simulink model "TWFL_V2"  (R2025b)
settings: Solver=daessc  StartTime=0.0  StopTime=15  RelTol=1e-3
values from neighbouring files (symbols this model uses):
  g = 9.81    [model_simplified.m]    (also in robotParams.m)
  g_fork = 2*pi*3    (= 18.8495559215)    [robotParams.m]
  g_lift = 2*pi*5    (= 31.4159265359)    [robotParams.m]
  g_reac = 2*pi*1    (= 6.28318530718)    [robotParams.m]
  Kd_fork = 100    [robotParams.m]
  Kd_lift = 50    [robotParams.m]
  Kp_fork = 200    [robotParams.m]
  Kp_lift = 200    [robotParams.m]
  Lx_b = 0.3    [robotParams.m]
  Lx_m = 0.1    [robotParams.m]
  Ly_b = 0.8    [robotParams.m]
  Ly_m = 0.3    [robotParams.m]
  Lz_b = 1    [robotParams.m]
  Lz_m = 1.5    [robotParams.m]
  M_arm_motor = 5    [robotParams.m]
  M_b = 16    [robotParams.m]
  M_fork_base = 2    [robotParams.m]
  M_m = 5    [robotParams.m]
  M_tooth = 1    [robotParams.m]
  M_w = 1    [robotParams.m]
  N = 40    [ocp_arm.m]    (also in ocp_simplified.m)
  r_w = 0.2    [model_simplified.m]    (also in robotParams.m)
  T_control = 1e-3    (= 0.001)    [robotParams.m]
  t_w = 0.05    [robotParams.m]
undefined symbols (not defined in the file or in its folder): dspblkCoreblockFVToolHelper, gcbh, Mn_33, Mn_44, X, Y, Z
libraries: sm_lib x49, nesl_utility x13, simulink x9, slpidlib x1, SignalEditorBlockLib x1
(part 1 of 3)
settings Model: Creator=oj  LastModifiedBy=angel
settings DataIOCC: SaveFormat=StructureWithTime
settings OptimizationCC: LifeSpan=inf
settings DebuggingCC: UnconnectedInputMsg=warning  UnconnectedOutputMsg=warning  UnconnectedLineMsg=warning  SFExecutionAtInitializationDiag=none  ArithmeticOperatorsInVariantConditions=warning
settings HardwareCC: ProdBitPerSizeT=32.0  ProdBitPerPtrDiffT=32.0  ProdWordSize=32.0  ProdHWDeviceType=Specified
settings SFSimCC: CustomCodeUndefinedFunction=UseInterfaceOnly
settings RTWCC: GPUComputeCapability=3.5
settings CodeAppCC: StateflowObjectComments=on

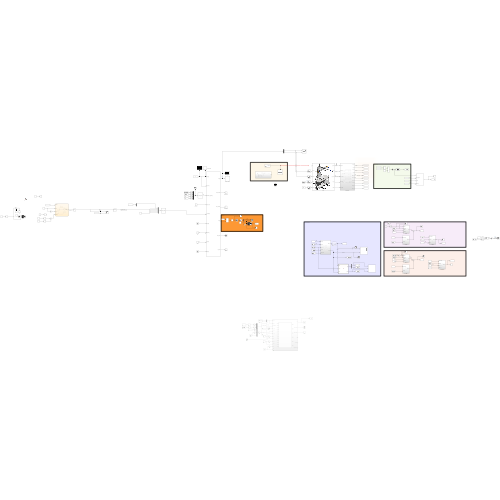
[thumbnail: Simulink's stored preview of the top-level diagram]
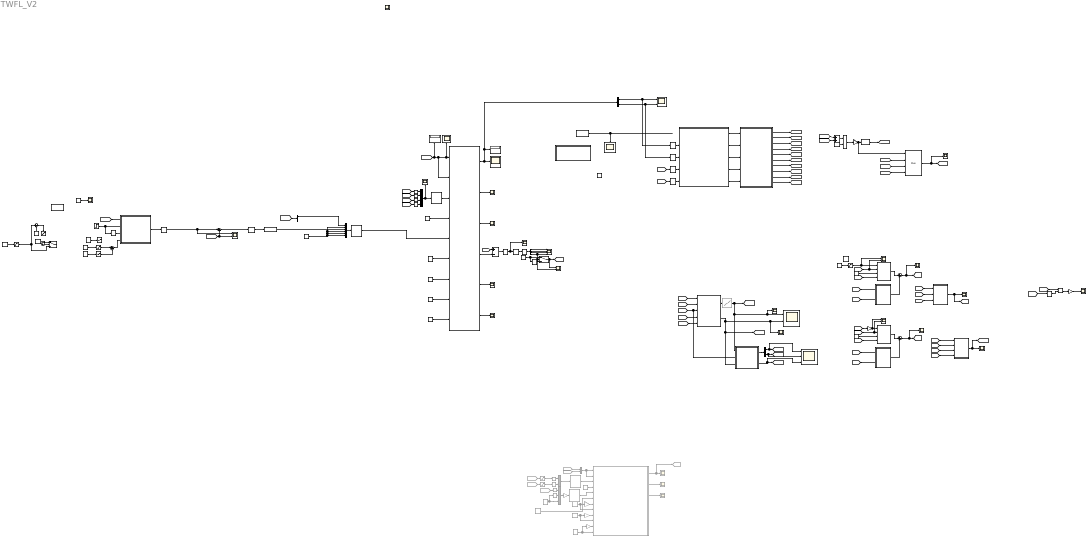
== system TWFL_V2 ==
  note: Collision
  note: CoG Estimation
  note: Calculations
  note: Disturbance
  note: FORK
  note: LIFT
  1-D Lookup Table2 : Lookup_n-D  Commented=through  NumberOfTableDimensions=1  BreakpointsForDimension1=[0:20]  Table=[0:20]  InterpMethod=Flat  InternalRulePriority=Speed  RndMeth=Simplest
  Abs : Abs  SaturateOnIntegerOverflow=off
  Abs1 : Abs  SaturateOnIntegerOverflow=off
  CPU : Scope
      settings: Description=status  ActiveDisplayYMinimum=0.0016298375  ActiveDisplayYMaximum=0.0033734625  DataLoggingVariableName=ScopeData3
  Calculations : Subsystem
  Chart : Stateflow chart  TreatAsAtomicUnit=on
  Clock1 : Clock
      settings: Decimation=9
  Constant{,16,42..43} (4 alike) : Constant  Value=0
  Constant14 : Constant
  Constant17 : Constant  Commented=on  Value=[0 0 0]
  Constant18 : Constant  Commented=on  Value=[0 0]
  Constant19 : Constant  Commented=on  Value=[pi/4; 0.5]
  Constant20 : Constant  Commented=on  Value=0
  Constant23 : Constant  Commented=on  Value=repmat([pi/4; 0.5],N-1,1)
  Constant26 : Constant  Commented=on  Value=repmat([100],N,1)
  Constant45 : Constant  Value=0.1
  Constant6 : Constant  Value=2
  Constant8 : Constant  Value=-2
  Cos : Trigonometry  Operator=cos
  Delay : Delay  DelayLength=1  InputProcessing=Columns as channels (frame based)
  Demux : Demux  Outputs=2
  Demux1 : Demux  Outputs=2
  Demux2 : Demux
  Demux4 : Demux
  Discrete Derivative : simulink/Discrete/Discrete Derivative  gainval=1.0  ICPrevScaledInput=0.0  OutMin=[]  OutMax=[]  OutDataType=fixdt(1, 16)  OutScaling=2^-10  DoSatur=off
  Discrete Derivative1 : simulink/Discrete/Discrete Derivative  gainval=1.0  ICPrevScaledInput=0.0  OutMin=[]  OutMax=[]  OutDataType=fixdt(1, 16)  OutScaling=2^-10  DoSatur=off
  Display2 : Display
  Divide : Product  Inputs=*/
  Divide1 : Product  Inputs=*/
  Fork DOB : Subsystem
  Fork RDOB : Subsystem
  From25 : From  Commented=on  GotoTag=pitch_pos
  From26 : From  Commented=on  GotoTag=dist_hat
  From5 : From  Commented=on  GotoTag=arm_pos
  From6 : From  Commented=on  GotoTag=arm_vel
  From7 : From  Commented=on  GotoTag=mass_hat
  Gain{,1,3..4} (4 alike) : Gain  Commented=on  Gain=-1
  Gain12 : Gain  Gain=1/g
  Gain18 : Gain  Gain=-1
  Gain2 : Gain  Gain=r_w
  Goto6 : Goto  Commented=on  GotoTag=torque_arm
  KKT residual : Scope
      settings: Description=status  ActiveDisplayYMinimum=-0.63612459745356664  ActiveDisplayYMaximum=2.0677690230743266  DataLoggingVariableName=ScopeData4
  Lift DOB : Subsystem
  Lift RDOB : Subsystem
  MATLAB Function1 : MATLAB Function  TreatAsAtomicUnit=on
  Mux : Mux
      settings: DisplayOption=signals
  Mux2 : Mux  Inputs=6
  Mux4 : Mux
  Mux6 : Mux  Commented=on  Inputs=2
  Mux7 : Mux  Commented=on  Inputs=2
  Mux8 : Mux  Commented=on  Inputs=3
  NOT : Logic  Operator=NOT  IconShape=distinctive  AllPortsSameDT=off  OutDataTypeStr=boolean
  NOT1 : Logic  Operator=NOT  IconShape=distinctive  AllPortsSameDT=off  OutDataTypeStr=boolean
  OCP status : Scope
      settings: Description=status  ActiveDisplayYMinimum=-0.0035735878879828986  ActiveDisplayYMaximum=2.0531825990917243
  PD fork : Subsystem
  PD lift : Subsystem
  PID Controller : slpidlib/PID Controller  Controller=PID  Form=Parallel  TimeDomain=Discrete-time  UseExternalTs=off  SampleTime=-1  IntegratorMethod=Forward Euler  FilterMethod=Forward Euler  ControllerParametersSource=internal  P=2  I=1  UseKiTs=off  D=0  UseExternalDerivativeSource=off  N=100  UseFilter=on  TunerSelectOption=Transfer Function Based (PID Tuner App)  InitialConditionSource=internal  InitialConditionForIntegrator=0  InitialConditionForFilter=0  DifferentiatorICPrevScaledInput=0  ExternalReset=none  TrackingMode=off  Kt=1  LimitOutput=off  SatLimitsSource=internal  UpperSaturationLimit=inf  LowerSaturationLimit=-inf  LinearizeAsGain=on  AntiWindupMode=none  Kb=1  LimitIntegrator=off  UpperIntegratorSaturationLimit=inf  LowerIntegratorSaturationLimit=-inf  POutMin=[]  POutMax=[]  IOutMin=[]  IOutMax=[]  DOutMin=[]  DOutMax=[]  NOutMin=[]  NOutMax=[]  SumOutMin=[]  SumOutMax=[]  SaturationOutMin=[]  SaturationOutMax=[]  PParamMin=[]  PParamMax=[]  IParamMin=[]  IParamMax=[]  DParamMin=[]  DParamMax=[]  NParamMin=[]  NParamMax=[]  KbParamMin=[]  KbParamMax=[]  KtParamMin=[]  KtParamMax=[]  KbOutMin=[]  KbOutMax=[]  KtOutMin=[]  KtOutMax=[]  IntegratorOutMin=[]  IntegratorOutMax=[]  FilterOutMin=[]  FilterOutMax=[]  SumI1OutMin=[]  SumI1OutMax=[]  SumI2OutMin=[]  SumI2OutMax=[]  SumI3OutMin=[]  SumI3OutMax=[]  SumI4OutMin=[]  SumI4OutMax=[]  SumDOutMin=[]  SumDOutMax=[]  DifferentiatorOutMin=[]  DifferentiatorOutMax=[]  FilterDiffOutCoefMin=[]  FilterDiffOutCoefMax=[]  ReciprocalOutMin=[]  ReciprocalOutMax=[]  SumDenOutMin=[]  SumDenOutMax=[]  SumNumOutMin=[]  SumNumOutMax=[]  DivideOutMin=[]  DivideOutMax=[]  UdiffTsProdOutMin=[]  UdiffTsProdOutMax=[]  NTsProdOutMin=[]  NTsProdOutMax=[]  UintegralTsProdOutMin=[]  UintegralTsProdOutMax=[]  UngainTsProdOutMin=[]  UngainTsProdOutMax=[]  ClampingZeroOutDataTypeStr=Inherit: Inherit via back propagation  ClampingZeroOutMin=[]  ClampingZeroOutMax=[]  FilterDenConstantOutDataTypeStr=Inherit: Inherit via back propagation  FilterDenConstantOutMin=[]  FilterDenConstantOutMax=[]  PCopyOutDataTypeStr=Inherit: Inherit via back propagation  PCopyOutMin=[]  PCopyOutMax=[]  NCopyOutDataTypeStr=Inherit: Inherit via back propagation  NCopyOutMin=[]  NCopyOutMax=[]  IntegratorContinuousStateAttributes=''  IntegratorStateMustResolveToSignalObject=off  IntegratorRTWStateStorageClass=Auto  FilterContinuousStateAttributes=''  FilterStateMustResolveToSignalObject=off  FilterRTWStateStorageClass=Auto  ParallelPVariant=InternalParameters  IdealPVariant=Disabled  IVariant=InternalParameters  DVariant=InternalParameters  IntegratorVariant=Discrete  SatVariant=Disabled  AWVariant=Passthrough  PCopyVariant=Disabled  TRVariant=Disabled  FdbkBlocksVariant=Forward  IdealPFdbkVariant=Disabled  SatFdbkVariant=Disabled  DerivativeFilterVariant=ForwardEulerFilter  NVariant=InternalParameters  NCopyVariant=Disabled  FilterICVariant=InternalICsFilter  IntegratorICVariant=InternalICs  ExternalResetVariant=Disabled  TRSumVariant=Passthrough  SumFdbkVariant=Disabled  SumVariant=Sum_PID  TsampFilterVariant=InternalTs  TsampNgainVariant=Passthrough  TsampIntegralVariant=Disabled_SignalSpec  ExternalSaturationOutDataTypeStr=Inherit: Same as second input  DerivativeSourceVariant=ErrorSignal  PreIntVariant=InternalPreInt
  Plant5 : Subsystem
      mask Display: image('plant.png');
  Push Button : PushButtonBlock  ButtonText=Start  ButtonType=Latch  IconOnColor=[0.0, 1.0, 0.0]  IconOffColor=[1.0, 1.0, 1.0]  IconColor=On  OffValue=0.000000
  Ramp1 : simulink/Sources/Ramp  slope=0.05  start=3  InitialOutput=0
  Ramp2 : simulink/Sources/Ramp  slope=1  start=9  InitialOutput=0
  Ramp3 : simulink/Sources/Ramp  slope=2  start=0  InitialOutput=0
  Ramp4 : simulink/Sources/Ramp  slope=1  start=1  InitialOutput=0
  Ramp5 : simulink/Sources/Ramp  slope=1  start=10  InitialOutput=0
  Ramp6 : simulink/Sources/Ramp  slope=1  start=5  InitialOutput=0
  Rate Transition{,1..3} (4 alike) : RateTransition  OutPortSampleTime=T_control
  S-Function1 : S-Function  FunctionName=acados_solver_sfunction_model_simplified  SFunctionDeploymentMode=off  EnableBusSupport=off
      mask Display:
      | % from the make_sfun file
      | global sfun_input_names sfun_output_names
      | for i = 1:length(sfun_input_names)
      | 	port_label('input', i, sfun_input_names{i})
      | end
      | for i = 1:length(sfun_output_names)
      | 	port_label('output', i, sfun_output_names{i})
      | end
  S-Function2 : S-Function  FunctionName=repmat_sfun  Parameters=N+1  SFunctionDeploymentMode=off  EnableBusSupport=off
  S-Function3 : S-Function  Commented=on  FunctionName=repmat_sfun  Parameters=N+1  SFunctionDeploymentMode=off  EnableBusSupport=off
  S-Function4 : S-Function  Commented=on  FunctionName=repmat_sfun  Parameters=N-1  SFunctionDeploymentMode=off  EnableBusSupport=off
  S-Function5 : S-Function  FunctionName=repmat_sfun  Parameters=N-1  SFunctionDeploymentMode=off  EnableBusSupport=off
  SQP iter : Scope
      settings: Description=status  ActiveDisplayYMinimum=-11.826905175074671  ActiveDisplayYMaximum=55.703090781193573  DataLoggingVariableName=ScopeData5
  Saturation : Saturate  UpperLimit=5  LowerLimit=0
  Saturation1 : Saturate
  Saturation2 : Saturate  UpperLimit=.25
  Saturation3 : Saturate
  Saturation4 : Saturate  Commented=on  UpperLimit=20  LowerLimit=0
  Saturation5 : Saturate  Commented=on  UpperLimit=0.6  LowerLimit=0.2
  Saturation6 : Saturate  UpperLimit=1  LowerLimit=0
  Saturation7 : Saturate  UpperLimit=1  LowerLimit=0
  Scope control : Scope
      settings: ActiveDisplayYMinimum=-179.76344795838239  ActiveDisplayYMaximum=28.261944980460278  DataLoggingVariableName=ScopeData6
  Scope state1 : Scope
      settings: ActiveDisplayYMinimum=-2.6646698598678142  ActiveDisplayYMaximum=0.29678375248917371  DataLoggingVariableName=ScopeData9
  Scope1 : Scope  NumInputPorts=4
      settings: ActiveDisplayYMinimum=-96.781255241402022  ActiveDisplayYMaximum=871.03129768928852  DataLoggingVariableName=ScopeData26
  Scope{2..3,10,12,17,26} (6 alike) : Scope  NumInputPorts=2
      Scope10 settings: ActiveDisplayYMinimum=-0.12499999999999997  ActiveDisplayYMaximum=1.125  DataLoggingVariableName=ScopeData28
      Scope12 settings: ActiveDisplayYMinimum=-1  ActiveDisplayYMaximum=1  DataLoggingVariableName=ScopeData31
      Scope17 settings: ActiveDisplayYMinimum=-1  ActiveDisplayYMaximum=1  DataLoggingVariableName=ScopeData35
      Scope2 settings: ActiveDisplayYMinimum=-4.7265728175160966  ActiveDisplayYMaximum=6.508300219679283  DataLoggingVariableName=ScopeData2
      Scope26 settings: ActiveDisplayYMinimum=0.31875  ActiveDisplayYMaximum=0.63125  DataLoggingVariableName=ScopeData32
      Scope3 settings: ActiveDisplayYMinimum=-12.49999999999882  ActiveDisplayYMaximum=12.499999999991127  DataLoggingVariableName=ScopeData10
  Scope{,4..7,9,11,16,18..21} (12 alike) : Scope
      Scope11 settings: ActiveDisplayYMinimum=-0.2386803915005089  ActiveDisplayYMaximum=1.7974378919712937  DataLoggingVariableName=ScopeData29
      Scope16 settings: ActiveDisplayYMinimum=-1  ActiveDisplayYMaximum=1  DataLoggingVariableName=ScopeData27
      Scope18 settings: ActiveDisplayYMinimum=-1  ActiveDisplayYMaximum=1  DataLoggingVariableName=ScopeData36
      Scope19 settings: ActiveDisplayYMinimum=-1  ActiveDisplayYMaximum=1  DataLoggingVariableName=ScopeData37
      Scope20 settings: ActiveDisplayYMinimum=74.24782414299321  ActiveDisplayYMaximum=93.660209670148674  DataLoggingVariableName=ScopeData39
      Scope21 settings: ActiveDisplayYMinimum=-1  ActiveDisplayYMaximum=1  DataLoggingVariableName=ScopeData40
      Scope4 settings: ActiveDisplayYMinimum=-125.68830085745365  ActiveDisplayYMaximum=62.810118223913989  DataLoggingVariableName=ScopeData11
      Scope5 settings: ActiveDisplayYMinimum=-7.37133327140659  ActiveDisplayYMaximum=14.471332987171895  DataLoggingVariableName=ScopeData12
      Scope6 settings: ActiveDisplayYMinimum=-0.193211762638459  ActiveDisplayYMaximum=0.32936826449448647  DataLoggingVariableName=ScopeData13
      Scope7 settings: ActiveDisplayYMinimum=-2.8032822197416674  ActiveDisplayYMaximum=3.1027732142135709  DataLoggingVariableName=ScopeData7
      Scope9 settings: ActiveDisplayYMinimum=-1  ActiveDisplayYMaximum=1  DataLoggingVariableName=ScopeData19
      Scope settings: ActiveDisplayYMinimum=-13.79726  ActiveDisplayYMaximum=10.28583
  Scope13 : Scope  Commented=on
      settings: ActiveDisplayYMinimum=-12.276347103940505  ActiveDisplayYMaximum=17.806393317198079  DataLoggingVariableName=ScopeData33
  Scope14 : Scope  Commented=on
      settings: ActiveDisplayYMinimum=-0.63087824577294693  ActiveDisplayYMaximum=5.157246754227053  DataLoggingVariableName=ScopeData34
  Scope15 : Scope  Commented=on
      settings: ActiveDisplayYMinimum=-1  ActiveDisplayYMaximum=1  DataLoggingVariableName=ScopeData38
  Scope8 : Scope  NumInputPorts=3
      settings: ActiveDisplayYMinimum=-8.2743101469477089  ActiveDisplayYMaximum=17.001393340631182  DataLoggingVariableName=ScopeData21
  Signal Generator : SignalGenerator  Units=rad/sec
  Signal Editor : SignalEditorBlockLib/Signal Editor  FileName=disturbance.mat  ActiveScenario=Scenario  ActiveSignal=Signal 1  IsBus=off  OutputBusObjectStr=Bus: BusObject  SampleTime=0  ZeroCross=off  OutputAfterFinalValue=Setting to zero  Unit=inherit  PreserveSignalName=on  ApplySigPropsToAllScenarios=on  ApplySigPropsToAllSignals=off  SignalPropertySource=Dialog parameters
  Signal Specification : SignalSpecification  OutDataTypeStr=double  Dimensions=1
  Signal Specification{1..4} (4 alike) : SignalSpecification  Dimensions=1
  Signal Specification{9..12} (4 alike) : SignalSpecification  Commented=on  Dimensions=1
  Step1 : Step  Time=5  SampleTime=0
  Subsystem : Subsystem
  Subsystem1 : Subsystem  Commented=on
  Subsystem2 : Subsystem
  Subtract : Sum  Inputs=+-
  Sum : Sum  Inputs=+|+
  Sum1 : Sum  Inputs=|+-
  Sum16 : Sum  Inputs=|++
  Sum17 : Sum  Inputs=|++
  Sum3 : Sum  Inputs=|+-
  Sum5 : Sum  Inputs=|+-
  Switch2 : Switch  Criteria=u2 > Threshold  Threshold=4.8  SaturateOnIntegerOverflow=off  InputSameDT=off
  Switch3 : Switch  Criteria=u2 > Threshold  Threshold=200  SaturateOnIntegerOverflow=off  InputSameDT=off
  lbu : Constant  Value=repmat([-10;-10],N,1)
  lbx : Constant  Value=repmat([-50; -pi/4; -3; -pi],N-1,1)
  q : Scope
      settings: ActiveDisplayYMinimum=-0.062737495046845726  ActiveDisplayYMaximum=0.56463747287082289  DataLoggingVariableName=ScopeData30
  u : Display
  ubu : Constant  Value=repmat([10;10],N,1)
  ubx : Constant  Value=repmat([500; pi/4; 5; pi],N-1,1)
  y_ref_0 : Constant  Value=zeros(1,6)
  wires:
  S-Function1/5 -> CPU/1
  S-Function1/6 -> SQP iter/1
  S-Function1/3 -> KKT residual/1
  Mux/1 -> Scope7/1, [q_0]  "x"
  S-Function1/4 -> Subtract/2
  S-Function1/2 -> OCP status/1
  S-Function1/1 -> Demux/1, u/1, Scope control/1  "u"
  lbx/1 -> S-Function1/6
  Demux/1 -> Rate Transition2/1, Scope3/1
  Calculations/1(rw_pos) -> [rw_pos]  "rw_angle"
  Calculations/3(lw_pos) -> [lw_pos]  "lw_angle"
  Calculations/5(pitch_pos) -> [pitch_pos]  "pitch_angle"
  Sum/1 -> Divide1/1
  Constant6/1 -> Divide1/2
  Divide1/1 -> Gain2/1
  Gain2/1 -> Mux/1, Discrete Derivative/1  "x"
  Discrete Derivative/1 -> [x_vel]  "x_dot"
  lbu/1 -> S-Function1/8
  ubu/1 -> S-Function1/9
  Demux/2 -> Rate Transition3/1, Scope3/2
  Mux2/1 -> S-Function5/1
  Demux2/1 -> Mux2/1
  Sum3/1 -> PID Controller/1
  Ramp3/1 -> Saturation1/1
  PID Controller/1 -> Signal Specification/1
  Signal Specification/1 -> Mux2/3
  ubx/1 -> S-Function1/7
  Ramp2/1 -> Sum5/2
  Clock1/1 -> Switch2/2
  Sum5/1 -> Saturation/1
  Chart/1(velocity_out) -> Delay/1  "reference_v"
  Calculations/4(lw_vel) -> [lw_vel]
  Calculations/9(arm_pos) -> [arm_pos]
  Calculations/8(lift_vel) -> [lift_vel]
  Plant5/5(armPos) -> Calculations/5(arm_angle)
  Plant5/4(lift_pos) -> Calculations/4(lift_height)
  Calculations/7(lift_pos) -> [lift_pos]
  Rate Transition1/1 -> Plant5/4(liftForce)
  [force_lift] -> Rate Transition1/1
  [arm_pos] -> Subsystem/4(arm_pos)
  Rate Transition/1 -> Plant5/5(armTorque)
  Plant5/3(pitch_angle) -> Calculations/3(pitch_angle)  "pitch_angle"
  Calculations/6(pitch_vel) -> [pitch_vel]
  Plant5/1(rw_angle) -> Calculations/1(rw_angle)  "rw_angle"
  Plant5/2(lw_angle) -> Calculations/2(lw_angle)  "lw_angle"
  [lift_pos] -> MATLAB Function1/2(pos_lift), Subsystem/3(lift_pos)
  Subsystem/1(mass_hat) -> 1-D Lookup Table2/1  "mass"
  Calculations/2(rw_vel) -> [rw_vel]
  [pitch_pos] -> Subsystem/2(pitch_pos)
  Calculations/10(arm_vel) -> [arm_vel]
  [torque_arm] -> Rate Transition/1
  Rate Transition2/1 -> Plant5/2(rwTorque)
  Rate Transition3/1 -> Plant5/3(lwTorque)
  MATLAB Function1/1(cdg) -> Demux1/1
  Demux1/1 -> Scope8/1, [cog_x]
  Demux1/2 -> Scope8/2, [cog_z]
  MATLAB Function1/2(I_total) -> Scope8/3, [inertia]
  [mass_hat] -> Signal Specification4/1
  [inertia] -> Signal Specification3/1
  [cog_x] -> Signal Specification2/1
  [cog_z] -> Signal Specification1/1
  Signal Specification1/1 -> Mux4/4
  Signal Specification2/1 -> Mux4/3
  Signal Specification3/1 -> Mux4/2
  Signal Specification4/1 -> Mux4/1
  Subsystem/2(dist_hat) -> [dist_hat], MATLAB Function1/3(d_hat), Scope18/1, Scope26/2  "distance"
  Sum17/1 -> Scope20/1, [force_lift]
  [pitch_pos] -> Gain18/1
  [lift_pos] -> Scope12/2, PD lift/2(posMeas)
  [force_lift] -> Lift DOB/1(Input Torque)
  Constant42/1 -> PD fork/3(velRef)
  Constant43/1 -> PD lift/3(velRef)
  Fork DOB/1(Est_dis) -> Sum16/2
  Lift DOB/1(Est_dis) -> Sum17/2
  [lift_vel] -> PD lift/4(velMeas)
  [torque_arm] -> Fork DOB/1(Input Torque)
  Sum16/1 -> Scope16/1, [torque_arm]
  PD lift/1(out) -> Sum17/1
  Ramp1/1 -> Saturation2/1
  [arm_vel] -> Fork DOB/2(Velocity)
  PD fork/1(out) -> Sum16/1
  Gain18/1 -> Scope17/1, PD fork/1(posRef)
  [arm_vel] -> PD fork/4(velMeas)
  [lift_vel] -> Lift DOB/2(Velocity)
  [arm_pos] -> Scope17/2, PD fork/2(posMeas)
  Subtract/1 -> Abs/1
  Abs/1 -> q/1, Discrete Derivative1/1
  Demux4/1 -> Scope1/1  "x_dot"
  Demux4/2 -> Scope1/2  "pitch_dot"
  Demux4/3 -> Scope1/3  "x_ddot"
  Demux4/4 -> Scope10/2, Switch3/2, Scope1/4  "pitch_ddot"
  Saturation1/1 -> Switch2/3, Sum5/1
  Constant8/1 -> Switch2/1
  Switch3/1 -> Scope10/1, [collision]
  [collision] -> Chart/1(collision)
  Step1/1 -> NOT/1, Chart/2(move)
  NOT/1 -> Chart/3(load)
  Delay/1 -> Scope2/1, Sum3/1
  Constant14/1 -> NOT1/1, Switch3/1
  NOT1/1 -> Switch3/3
  Discrete Derivative1/1 -> Abs1/1
  Constant16/1 -> Scope11/1
  Ramp4/1 -> Saturation3/1
  Mux6/1 -> Subsystem1/2(ubx_0), Subsystem1/1(lbx_0)
  From5/1 -> Mux6/1
  From6/1 -> Mux6/2
  Signal Specification9/1 -> Mux7/2
  Mux7/1 -> S-Function3/1
  From7/1 -> Saturation4/1
  Signal Specification12/1 -> Mux7/1
  From26/1 -> Saturation5/1
  S-Function3/1 -> Subsystem1/3(parameters)
  Constant17/1 -> Subsystem1/4(y_ref_0)
  S-Function4/1 -> Subsystem1/5(y_ref)
  Constant20/1 -> Signal Specification11/1, Mux8/3
  Signal Specification10/1 -> Mux8/1
  From25/1 -> Signal Specification10/1
  Mux8/1 -> Gain/1
  Signal Specification11/1 -> Mux8/2
  Gain/1 -> S-Function4/1
  Constant18/1 -> Subsystem1/6(y_ref_e)
  Gain1/1 -> Subsystem1/7(lbx)
  Constant23/1 -> Subsystem1/8(ubx), Gain1/1
  Constant19/1 -> Subsystem1/10(ubx_e), Gain3/1
  Gain3/1 -> Subsystem1/9(lbx_e)
  Subsystem1/2(solver status) -> Scope14/1
  Subsystem1/3(KKT residual) -> Scope15/1
  Gain4/1 -> Subsystem1/11(lbu)
  Constant26/1 -> Gain4/1, Subsystem1/12(ubu)
  Subsystem1/1(u0) -> Goto6/1, Scope13/1
  Saturation4/1 -> Signal Specification12/1
  Saturation5/1 -> Signal Specification9/1
  Mux4/1 -> S-Function2/1, Scope19/1
  1-D Lookup Table2/1 -> [mass_hat], Scope21/1, Scope26/1, MATLAB Function1/1(m_hat)  "mass"
  Signal Editor/1 -> Scope5/1
  [lw_pos] -> Sum/2
  [rw_pos] -> Sum/1
  [pitch_pos] -> Mux/2
  [pitch_vel] -> Mux/4
  [x_vel] -> Mux/3
  [q_0] -> Subtract/1
  [q_0] -> Demux2/1
  [q_0] -> Display2/1, S-Function1/2, Scope state1/1, S-Function1/1  "x"
  y_ref_0/1 -> S-Function1/4
  Constant/1 -> Mux2/6, Mux2/5, Mux2/4, Mux2/2
  [x_vel] -> Scope2/2, Sum3/2
  [force_lift] -> Lift RDOB/1(Input Torque)
  [lift_vel] -> Lift RDOB/2(Velocity)
  [pitch_pos] -> Lift RDOB/3(Pitch)
  Lift RDOB/1(Est_dis) -> [external_lift], Scope4/1
  Cos/1 -> Divide/2
  Divide/1 -> Gain12/1
  [external_lift] -> Divide/1
  [pitch_pos] -> Cos/1
  Gain12/1 -> Scope6/1  "Estimated ml"
  [pitch_pos] -> Fork RDOB/3(pitch_pos)
  [torque_arm] -> Fork RDOB/1(Input Torque)
  [arm_vel] -> Fork RDOB/2(Velocity)
  [arm_pos] -> Fork RDOB/4(arm_pos)
  Fork RDOB/1(Est_dis) -> [external_fork], Scope9/1
  [external_lift] -> Subsystem/1(force_lift)
  [external_fork] -> Subsystem/5(torque_arm)
  Abs1/1 -> Demux4/1
  Saturation2/1 -> PD lift/1(posRef), Scope12/1
  Sum1/1 -> Chart/4(velocity_in)
  Saturation6/1 -> Sum1/2
  Ramp6/1 -> Saturation7/1
  Ramp5/1 -> Saturation6/1
  Saturation7/1 -> Sum1/1
  S-Function2/1 -> S-Function1/3
  S-Function5/1 -> S-Function1/5

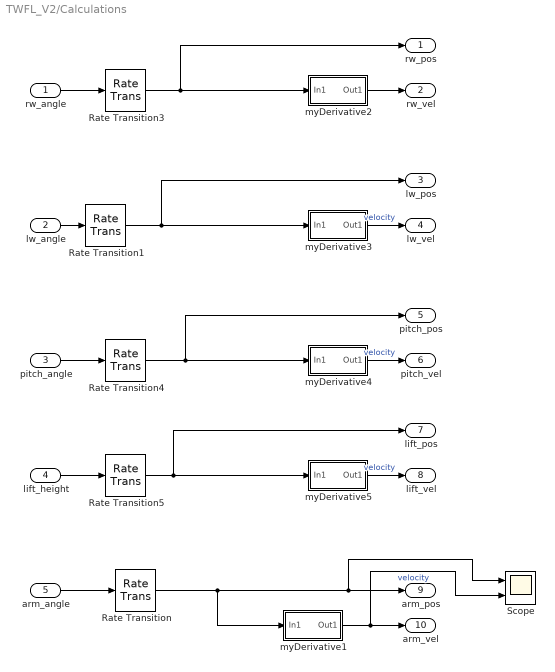
== system TWFL_V2/Calculations ==
  rw_angle : Inport
  lw_angle : Inport  Port=2
  pitch_angle : Inport  Port=3
  lift_height : Inport  Port=4
  arm_angle : Inport  Port=5
  Rate Transition{,1,3..5} (5 alike) : RateTransition  OutPortSampleTime=T_control
  Scope : Scope  NumInputPorts=2
      settings: ActiveDisplayYMinimum=-0.3840409140605956  ActiveDisplayYMaximum=2.1541582270060031  DataLoggingVariableName=ScopeData22
  myDerivative1 : Subsystem
      mask Display: image('myDerivative.png');
  myDerivative2 : Subsystem
      mask Display: image('myDerivative.png');
  myDerivative3 : Subsystem
      mask Display: image('myDerivative.png');
  myDerivative4 : Subsystem
      mask Display: image('myDerivative.png');
  myDerivative5 : Subsystem
      mask Display: image('myDerivative.png');
  rw_pos : Outport
  rw_vel : Outport  Port=2
  lw_pos : Outport  Port=3
  lw_vel : Outport  Port=4
  pitch_pos : Outport  Port=5
  pitch_vel : Outport  Port=6
  lift_pos : Outport  Port=7
  lift_vel : Outport  Port=8
  arm_pos : Outport  Port=9
  arm_vel : Outport  Port=10
  wires:
  rw_angle/1 -> Rate Transition3/1
  lw_angle/1 -> Rate Transition1/1
  pitch_angle/1 -> Rate Transition4/1
  Rate Transition5/1 -> myDerivative5/1(In1), lift_pos/1
  myDerivative2/1(Out1) -> rw_vel/1
  myDerivative3/1(Out1) -> lw_vel/1  "velocity"
  myDerivative4/1(Out1) -> pitch_vel/1  "velocity"
  myDerivative5/1(Out1) -> lift_vel/1  "velocity"
  lift_height/1 -> Rate Transition5/1
  arm_angle/1 -> Rate Transition/1
  myDerivative1/1(Out1) -> Scope/2, arm_vel/1  "velocity"
  Rate Transition/1 -> myDerivative1/1(In1), Scope/1, arm_pos/1
  Rate Transition1/1 -> myDerivative3/1(In1), lw_pos/1
  Rate Transition3/1 -> myDerivative2/1(In1), rw_pos/1
  Rate Transition4/1 -> myDerivative4/1(In1), pitch_pos/1

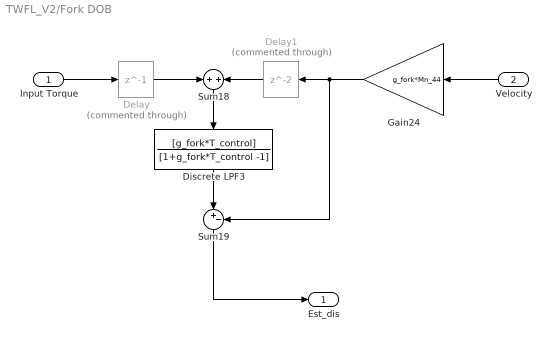
== system TWFL_V2/Fork DOB ==
  Input Torque : Inport
  Velocity : Inport  Port=2
  Delay : Delay  Commented=through  DelayLength=1  InputProcessing=Columns as channels (frame based)  SampleTime=T_control
  Delay1 : Delay  Commented=through  InputProcessing=Columns as channels (frame based)  SampleTime=T_control
  Discrete LPF3 : DiscreteFilter  LoadFcn=dspblkCoreblockFVToolHelper(gcbh,'load');  Numerator=[g_fork*T_control]  Denominator=[1+g_fork*T_control -1]
      settings: CopyFcn=dspblkCoreblockFVToolHelper(gcbh,'copy');  DeleteFcn=dspblkCoreblockFVToolHelper(gcbh,'close');  ModelCloseFcn=dspblkCoreblockFVToolHelper(gcbh,'close');  PreSaveFcn=dspblkCoreblockFVToolHelper(gcbh,'presave');  PostSaveFcn=dspblkCoreblockFVToolHelper(gcbh,'postsave');  CloseFcn=dspblkCoreblockFVToolHelper(gcbh,'close');
  Gain24 : Gain  Gain=g_fork*Mn_44
  Sum18 : Sum  Inputs=+|+
  Sum19 : Sum  Inputs=|+-
  Est_dis : Outport
  wires:
  Delay/1 -> Sum18/1
  Sum19/1 -> Est_dis/1
  Velocity/1 -> Gain24/1
  Input Torque/1 -> Delay/1
  Sum18/1 -> Discrete LPF3/1
  Gain24/1 -> Sum19/2, Delay1/1
  Discrete LPF3/1 -> Sum19/1
  Delay1/1 -> Sum18/2

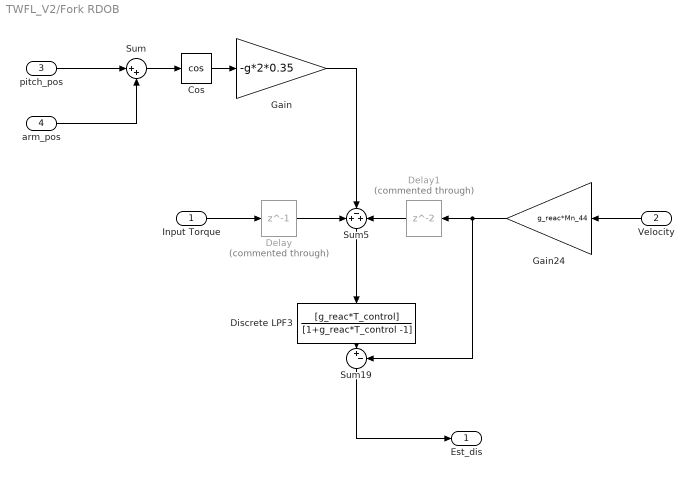
== system TWFL_V2/Fork RDOB ==
  Input Torque : Inport
  Velocity : Inport  Port=2
  pitch_pos : Inport  Port=3
  arm_pos : Inport  Port=4
  Cos : Trigonometry  Operator=cos
  Delay : Delay  Commented=through  DelayLength=1  InputProcessing=Columns as channels (frame based)  SampleTime=T_control
  Delay1 : Delay  Commented=through  InputProcessing=Columns as channels (frame based)  SampleTime=T_control
  Discrete LPF3 : DiscreteFilter  LoadFcn=dspblkCoreblockFVToolHelper(gcbh,'load');  Numerator=[g_reac*T_control]  Denominator=[1+g_reac*T_control -1]
      settings: CopyFcn=dspblkCoreblockFVToolHelper(gcbh,'copy');  DeleteFcn=dspblkCoreblockFVToolHelper(gcbh,'close');  ModelCloseFcn=dspblkCoreblockFVToolHelper(gcbh,'close');  PreSaveFcn=dspblkCoreblockFVToolHelper(gcbh,'presave');  PostSaveFcn=dspblkCoreblockFVToolHelper(gcbh,'postsave');  CloseFcn=dspblkCoreblockFVToolHelper(gcbh,'close');
  Gain : Gain  Gain=-g*2*0.35
  Gain24 : Gain  Gain=g_reac*Mn_44
  Sum : Sum  Inputs=|++
  Sum19 : Sum  Inputs=|+-
  Sum5 : Sum  Inputs=+-+
  Est_dis : Outport
  wires:
  Delay1/1 -> Sum5/3
  Discrete LPF3/1 -> Sum19/1
  Gain24/1 -> Delay1/1, Sum19/2
  Sum5/1 -> Discrete LPF3/1
  Input Torque/1 -> Delay/1
  Velocity/1 -> Gain24/1
  Sum19/1 -> Est_dis/1
  Delay/1 -> Sum5/1
  Sum/1 -> Cos/1
  Cos/1 -> Gain/1
  pitch_pos/1 -> Sum/1
  arm_pos/1 -> Sum/2
  Gain/1 -> Sum5/2

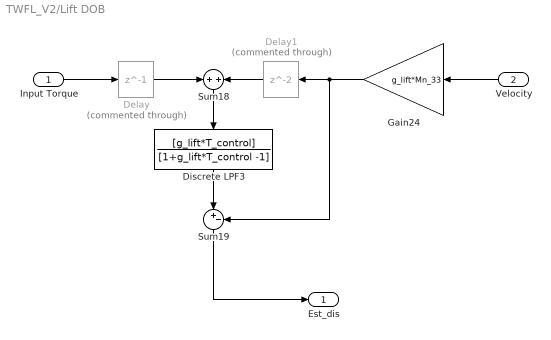
== system TWFL_V2/Lift DOB ==
  Input Torque : Inport
  Velocity : Inport  Port=2
  Delay : Delay  Commented=through  DelayLength=1  InputProcessing=Columns as channels (frame based)  SampleTime=T_control
  Delay1 : Delay  Commented=through  InputProcessing=Columns as channels (frame based)  SampleTime=T_control
  Discrete LPF3 : DiscreteFilter  LoadFcn=dspblkCoreblockFVToolHelper(gcbh,'load');  Numerator=[g_lift*T_control]  Denominator=[1+g_lift*T_control -1]
      settings: CopyFcn=dspblkCoreblockFVToolHelper(gcbh,'copy');  DeleteFcn=dspblkCoreblockFVToolHelper(gcbh,'close');  ModelCloseFcn=dspblkCoreblockFVToolHelper(gcbh,'close');  PreSaveFcn=dspblkCoreblockFVToolHelper(gcbh,'presave');  PostSaveFcn=dspblkCoreblockFVToolHelper(gcbh,'postsave');  CloseFcn=dspblkCoreblockFVToolHelper(gcbh,'close');
  Gain24 : Gain  Gain=g_lift*Mn_33
  Sum18 : Sum  Inputs=+|+
  Sum19 : Sum  Inputs=|+-
  Est_dis : Outport
  wires:
  Delay1/1 -> Sum18/2
  Discrete LPF3/1 -> Sum19/1
  Gain24/1 -> Delay1/1, Sum19/2
  Sum18/1 -> Discrete LPF3/1
  Input Torque/1 -> Delay/1
  Velocity/1 -> Gain24/1
  Sum19/1 -> Est_dis/1
  Delay/1 -> Sum18/1

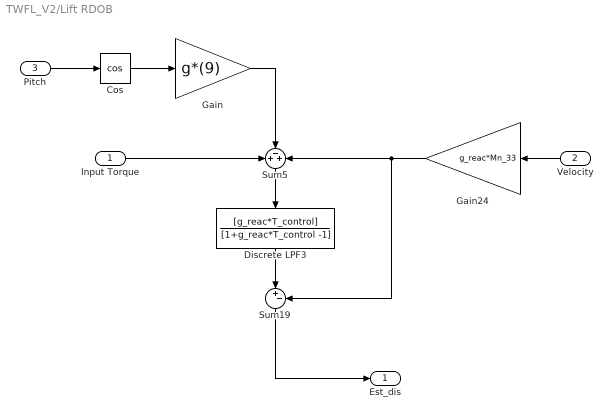
== system TWFL_V2/Lift RDOB ==
  Input Torque : Inport
  Velocity : Inport  Port=2
  Pitch : Inport  Port=3
  Cos : Trigonometry  Operator=cos
  Discrete LPF3 : DiscreteFilter  LoadFcn=dspblkCoreblockFVToolHelper(gcbh,'load');  Numerator=[g_reac*T_control]  Denominator=[1+g_reac*T_control -1]
      settings: CopyFcn=dspblkCoreblockFVToolHelper(gcbh,'copy');  DeleteFcn=dspblkCoreblockFVToolHelper(gcbh,'close');  ModelCloseFcn=dspblkCoreblockFVToolHelper(gcbh,'close');  PreSaveFcn=dspblkCoreblockFVToolHelper(gcbh,'presave');  PostSaveFcn=dspblkCoreblockFVToolHelper(gcbh,'postsave');  CloseFcn=dspblkCoreblockFVToolHelper(gcbh,'close');
  Gain : Gain  Gain=g*(9)
  Gain24 : Gain  Gain=g_reac*Mn_33
  Sum19 : Sum  Inputs=|+-
  Sum5 : Sum  Inputs=+-+
  Est_dis : Outport
  wires:
  Input Torque/1 -> Sum5/1
  Sum19/1 -> Est_dis/1
  Velocity/1 -> Gain24/1
  Sum5/1 -> Discrete LPF3/1
  Discrete LPF3/1 -> Sum19/1
  Gain24/1 -> Sum5/3, Sum19/2
  Pitch/1 -> Cos/1
  Cos/1 -> Gain/1
  Gain/1 -> Sum5/2

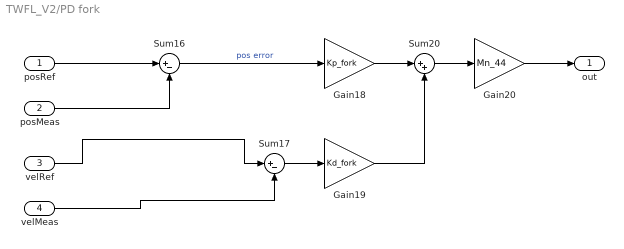
== system TWFL_V2/PD fork ==
  posRef : Inport
  posMeas : Inport  Port=2
  velRef : Inport  Port=3
  velMeas : Inport  Port=4
  Gain18 : Gain  Gain=Kp_fork
  Gain19 : Gain  Gain=Kd_fork
  Gain20 : Gain  Gain=Mn_44
  Sum16 : Sum  Inputs=|+-
  Sum17 : Sum  Inputs=|+-
  Sum20 : Sum  Inputs=|++
  out : Outport
  wires:
  Sum16/1 -> Gain18/1  "pos error"
  Gain18/1 -> Sum20/1
  Sum17/1 -> Gain19/1
  posRef/1 -> Sum16/1
  Sum20/1 -> Gain20/1
  Gain19/1 -> Sum20/2
  Gain20/1 -> out/1
  posMeas/1 -> Sum16/2
  velRef/1 -> Sum17/1
  velMeas/1 -> Sum17/2

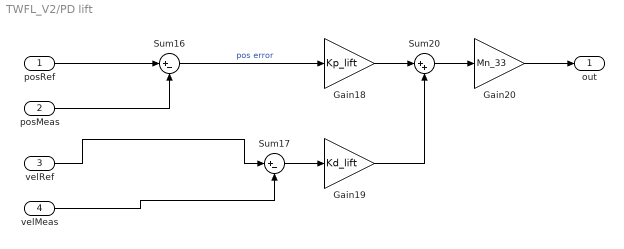
== system TWFL_V2/PD lift ==
  posRef : Inport
  posMeas : Inport  Port=2
  velRef : Inport  Port=3
  velMeas : Inport  Port=4
  Gain18 : Gain  Gain=Kp_lift
  Gain19 : Gain  Gain=Kd_lift
  Gain20 : Gain  Gain=Mn_33
  Sum16 : Sum  Inputs=|+-
  Sum17 : Sum  Inputs=|+-
  Sum20 : Sum  Inputs=|++
  out : Outport
  wires:
  velMeas/1 -> Sum17/2
  velRef/1 -> Sum17/1
  posMeas/1 -> Sum16/2
  Gain20/1 -> out/1
  Gain19/1 -> Sum20/2
  Sum20/1 -> Gain20/1
  posRef/1 -> Sum16/1
  Sum17/1 -> Gain19/1
  Gain18/1 -> Sum20/1
  Sum16/1 -> Gain18/1  "pos error"
